simulink model "pll_fast_model"  (R2023a)
settings: Solver=VariableStepAuto  StartTime=0.0  StopTime=0.03  RelTol=1e-3
values from neighbouring files (symbols this model uses):
  t_ADC = 1/f_ADC    (= 2e-05)    [uz_ssi_interface_init.m]
  t_clock = 1/f_clock    (= 1e-08)    [uz_ssi_interface_init.m]
undefined symbols (not defined in the file or in its folder): PLL
libraries: hdlsllib x2, simulink x1
settings Model: Creator=micha  LastModifiedBy=micha

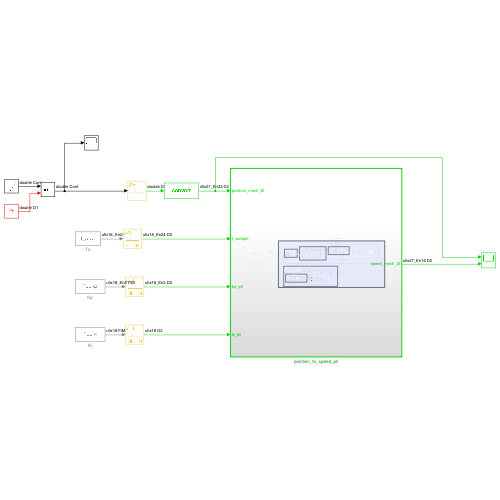
[thumbnail: Simulink's stored preview of the top-level diagram]
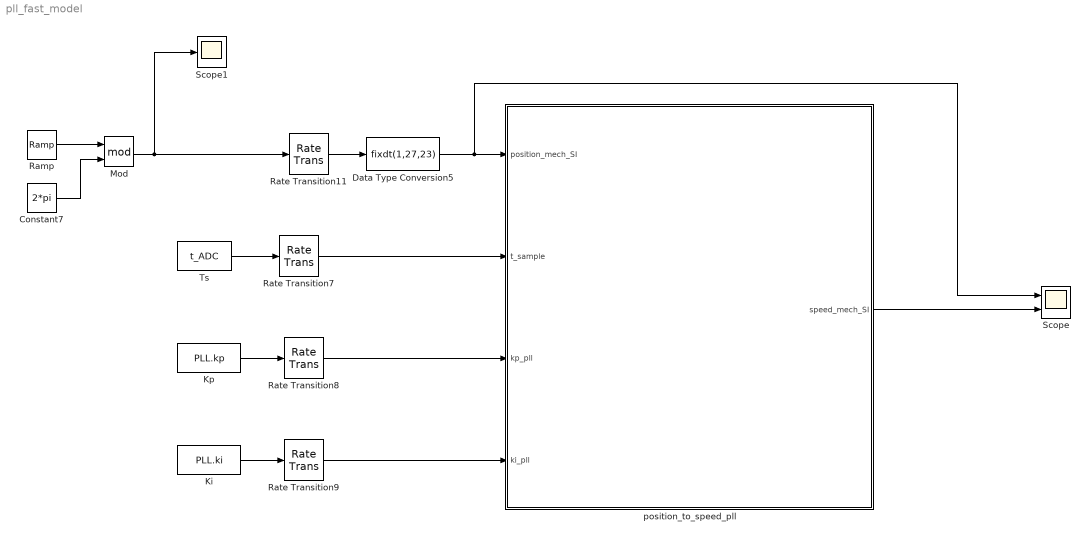
== system pll_fast_model ==
  Constant7 : Constant  Value=2*pi  SampleTime=t_clock
  Data Type Conversion5 : DataTypeConversion  OutDataTypeStr=fixdt(1,27,23)  SaturateOnIntegerOverflow=off  RndMeth=Floor
  Ki : Constant  Value=PLL.ki  OutDataTypeStr=fixdt(0,18,0)  SampleTime=-1
  Kp : Constant  Value=PLL.kp  OutDataTypeStr=fixdt(0,18,5)  SampleTime=-1
  Mod : Math  Operator=mod
  Ramp : simulink/Sources/Ramp  slope=-2*pi*100  start=7.5e-5  InitialOutput=0
  Rate Transition{7..9,11} (4 alike) : RateTransition  OutPortSampleTime=t_ADC
  Scope : Scope  NumInputPorts=2
  Scope1 : Scope
  Ts : Constant  Value=t_ADC  OutDataTypeStr=fixdt(0,18,24)  SampleTime=-1
  position_to_speed_pll : Subsystem  TreatAsAtomicUnit=on
      settings: LibrarySourceBlock=|
      | hdlsllib/Ports &
      | Subsystems/Triggered
      | Subsystem
  wires:
  Ramp/1 -> Mod/1
  Rate Transition11/1 -> Data Type Conversion5/1
  Constant7/1 -> Mod/2
  Data Type Conversion5/1 -> Scope/1, position_to_speed_pll/1(position_mech_SI)
  Ts/1 -> Rate Transition7/1
  Rate Transition7/1 -> position_to_speed_pll/2(t_sample)
  Rate Transition8/1 -> position_to_speed_pll/3(kp_pll)
  Rate Transition9/1 -> position_to_speed_pll/4(ki_pll)
  Kp/1 -> Rate Transition8/1
  Ki/1 -> Rate Transition9/1
  position_to_speed_pll/1(speed_mech_SI) -> Scope/2
  Mod/1 -> Scope1/1, Rate Transition11/1

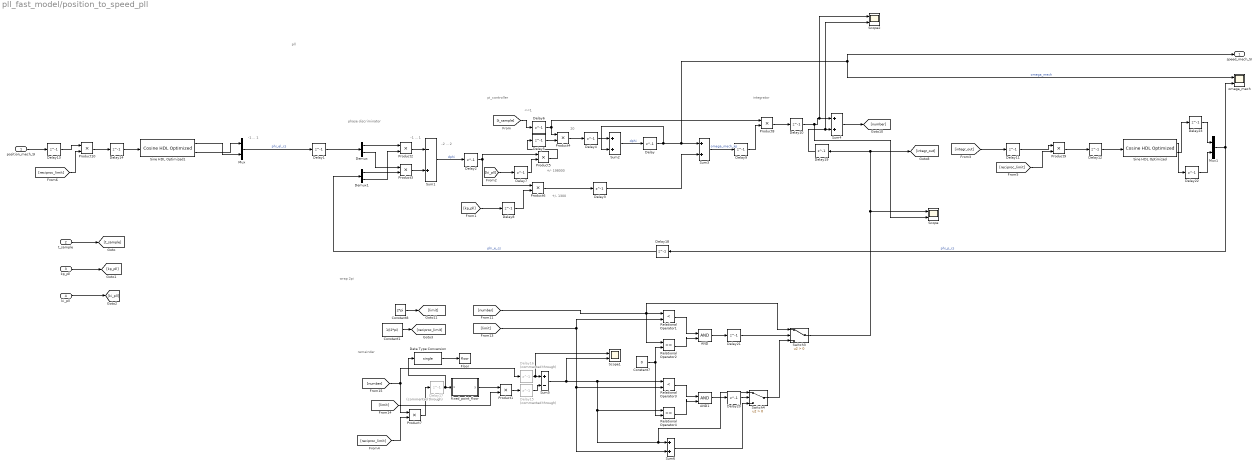
== system pll_fast_model/position_to_speed_pll ==
  note: remainder
  note: +/- 1300
  note: 20
  note: integrator
  note: -1 ... 1
  note: pll
  note: -1 ... 1
  note: phase discriminator
  note: <<1
  note: wrap 2pi
  note: -2 ... 2
  note: +/- 198000
  note: pi_controller
  position_mech_SI : Inport
  t_sample : Inport  Port=2
  kp_pll : Inport  Port=3
  ki_pll : Inport  Port=4
  AND : Logic  IconShape=distinctive  AllPortsSameDT=off  OutDataTypeStr=boolean
  AND1 : Logic  IconShape=distinctive  AllPortsSameDT=off  OutDataTypeStr=boolean
  Constant1 : Constant  Value=1/(2*pi)  OutDataTypeStr=fixdt(0,18,20)  SampleTime=-1
  Constant7 : Constant  Value=0  OutDataTypeStr=fixdt(0,27,24)  SampleTime=-1
  Constant8 : Constant  Value=2*pi  OutDataTypeStr=fixdt(0,18,15)  SampleTime=-1
  Data Type Conversion : DataTypeConversion  OutDataTypeStr=single  SaturateOnIntegerOverflow=off  RndMeth=Floor
  Delay{,19..23} (6 alike) : Delay  DelayLength=1
  Delay1 : Delay  DelayLength=1  InitialCondition=[1 0]
  Delay{2..14} (13 alike) : Delay  DelayLength=1  InitialCondition=0
  Delay15 : Delay  Commented=through  DelayLength=1  InitialCondition=0
  Delay16 : Delay  Commented=through  DelayLength=1  InitialCondition=0
  Delay17 : Delay  Commented=through  DelayLength=1  InitialCondition=0
  Delay18 : Delay  DelayLength=1  InitialCondition=[1 0]
  Demux : Demux  Outputs=2
  Demux1 : Demux  Outputs=2
  Floor : Rounding
  Mux : Mux  Inputs=2
  Mux1 : Mux  Inputs=2
  Product1 : Product  OutDataTypeStr=fixdt(1,27,23)
  Product10 : Product  OutDataTypeStr=fixdt(1,27,20)
  Product2 : Product  OutDataTypeStr=fixdt(1,27,25)
  Product3 : Product  OutDataTypeStr=fixdt(1,27,25)
  Product4 : Product  OutDataTypeStr=fixdt(1,27,20)
  Product5 : Product  OutDataTypeStr=fixdt(1,27,8)
  Product6 : Product  OutDataTypeStr=fixdt(1,27,14)
  Product7 : Product  OutDataTypeStr=fixdt(1,27,23)
  Product8 : Product  OutDataTypeStr=fixdt(1,27,26)
  Product9 : Product  OutDataTypeStr=fixdt(1,27,20)
  Relational Operator1 : RelationalOperator  Operator=<  OutDataTypeStr=boolean  RndMeth=Simplest  InputSameDT=off
  Relational Operator2 : RelationalOperator  OutDataTypeStr=boolean  RndMeth=Simplest  InputSameDT=off
  Relational Operator3 : RelationalOperator  Operator=<  OutDataTypeStr=boolean  RndMeth=Simplest  InputSameDT=off
  Relational Operator4 : RelationalOperator  OutDataTypeStr=boolean  RndMeth=Simplest  InputSameDT=off
  Scope : Scope  NumInputPorts=2
  Scope1 : Scope  NumInputPorts=2
  Scope2 : Scope  NumInputPorts=2
  Sine HDL Optimized : hdlsllib/Lookup Tables/Cosine HDL Optimized  OutputFormula=sin(2*pi*u) and cos(2*pi*u)  NumDataPoints=256  TableDataTypeStr=fixdt(0,26,20)  SimulateLUTROMDelay=off
      settings: LibrarySourceBlock=|
      | hdlsllib/Lookup
      | Tables/Sine
      | HDL Optimized
  Sine HDL Optimized1 : hdlsllib/Lookup Tables/Cosine HDL Optimized  OutputFormula=sin(2*pi*u) and cos(2*pi*u)  NumDataPoints=256  TableDataTypeStr=fixdt(0,26,20)  SimulateLUTROMDelay=off
      settings: LibrarySourceBlock=|
      | hdlsllib/Lookup
      | Tables/Sine
      | HDL Optimized
  Sum1 : Sum  Inputs=-+  AccumDataTypeStr=fixdt(1,27,24)
  Sum2 : Sum  OutDataTypeStr=fixdt(1,27,16)
  Sum3 : Sum  OutDataTypeStr=fixdt(1,27,14)
  Sum4 : Sum  OutDataTypeStr=fixdt(1,27,23)
  Sum5 : Sum  Inputs=+-  OutDataTypeStr=fixdt(1,27,23)
  Sum6 : Sum  OutDataTypeStr=fixdt(1,27,23)
  Switch3 : Switch  Criteria=u2 > Threshold  SaturateOnIntegerOverflow=off  InputSameDT=off
  Switch4 : Switch  Criteria=u2 > Threshold  SaturateOnIntegerOverflow=off  InputSameDT=off
  fixed_point_floor : MATLAB Function  TreatAsAtomicUnit=on
  omega_mech : Scope  NumInputPorts=2
  speed_mech_SI : Outport  InitialOutput=[0]
  wires:
  Product2/1 -> Sum1/1
  Constant8/1 -> [limit]
  Delay19/1 -> Sum4/2, Scope2/2
  Demux/1 -> Product2/1
  Mux1/1 -> omega_mech/2, Delay18/1  "phi_p_cs"
  [ki_pll] -> Delay7/1
  Sine HDL Optimized/2 -> Delay23/1
  Sum3/1 -> Delay9/1  "omega_mech_kp"
  Demux1/2 -> Product2/2
  Switch3/1 -> Scope/1, Delay19/1, [integr_out]
  Product3/1 -> Sum1/2
  Product4/1 -> Delay4/1
  Delay/1 -> speed_mech_SI/1, omega_mech/1, Sum3/1, Sum2/2  "omega_mech"
  Product8/1 -> Delay10/1
  [limit] -> Product1/2
  Switch4/1 -> Switch3/3
  [integr_out] -> Delay11/1
  Product1/1 -> Delay15/1
  Relational Operator3/1 -> AND1/1
  Product9/1 -> Delay12/1
  [number] -> Relational Operator2/1, Switch3/1, Relational Operator1/1
  Relational Operator2/1 -> AND/2
  Sum4/1 -> [number]
  Sum1/1 -> Delay2/1  "dphi"
  [limit] -> Relational Operator1/2, Sum6/2, Relational Operator3/2
  Product5/1 -> Delay5/1
  Product10/1 -> Delay14/1
  [number] -> Product7/1, Delay16/1
  Demux/2 -> Product3/1
  Delay6/1 -> Product4/1, Product8/1
  Demux1/1 -> Product3/2
  Delay18/1 -> Demux1/1  "phi_e_cs"
  Sine HDL Optimized/1 -> Delay22/1
  Mux/1 -> Delay1/1  "phi_el_cs"
  Relational Operator1/1 -> AND/1
  Product6/1 -> Delay3/1
  [kp_pll] -> Delay8/1
  AND/1 -> Delay21/1
  Sine HDL Optimized1/1 -> Mux/2
  Product7/1 -> Delay17/1
  Sum2/1 -> Delay/1  "dphi"
  Sum6/1 -> Switch4/3
  Sine HDL Optimized1/2 -> Mux/1
  Relational Operator4/1 -> AND1/2
  AND1/1 -> Delay20/1
  fixed_point_floor/1(y) -> Product1/1
  position_mech_SI/1 -> Delay13/1
  Constant7/1 -> Relational Operator2/2, Relational Operator4/2
  t_sample/1 -> [t_sample]
  kp_pll/1 -> [kp_pll]
  ki_pll/1 -> [ki_pll]
  Delay1/1 -> Demux/1
  Delay2/1 -> Product5/1, Product6/1
  Delay3/1 -> Sum3/2
  Delay4/1 -> Sum2/1
  Delay5/1 -> Product4/2
  Delay7/1 -> Product5/2
  Delay8/1 -> Product6/2
  Delay9/1 -> Product8/2
  [t_sample] -> Delay6/1
  Delay10/1 -> Scope/2, Scope2/1, Sum4/1
  Delay11/1 -> Product9/1
  Delay12/1 -> Sine HDL Optimized/1
  Delay13/1 -> Product10/1
  Delay14/1 -> Sine HDL Optimized1/1
  Delay15/1 -> Sum5/2
  Delay16/1 -> Scope1/1, Sum5/1
  Delay17/1 -> Data Type Conversion/1, fixed_point_floor/1(x)
  Sum5/1 -> Scope1/2, Switch4/1, Sum6/1, Relational Operator4/1, Relational Operator3/1
  Constant1/1 -> [reciproc_limit]
  [reciproc_limit] -> Product7/2
  Delay20/1 -> Switch4/2
  Delay21/1 -> Switch3/2
  [reciproc_limit] -> Product9/2
  [reciproc_limit] -> Product10/2
  Delay22/1 -> Mux1/2
  Delay23/1 -> Mux1/1
  Data Type Conversion/1 -> Floor/1

== matlab function pll_fast_model/position_to_speed_pll/fixed_point_floor ==
  data: x input; y output
function y = fcn(x)
%#codegen
x_floor = bitsra(x, x.FractionLength);  % Shift right to remove fraction
x_floor = bitsll(x_floor, x.FractionLength);  % Shift left to restore scale

y = x_floor;
